simulink model "SC_FFNN_trainlm_10_10_10_10_Dec_8_M"  (R2021a)
settings: Solver=VariableStepAuto  StartTime=0.0  StopTime=35  FixedStep=0.1  MaxStep=.1  RelTol=1e-3
model workspace (MAT data in the model file):
  T = [0 0.05 0.1 0.15 0.2 0.25 0.3 0.35 0.4 0.45 0.5 0.55 ... (701 elements, 701x1)]
  U = [3.99594136536 3.99594136536 3.99594136536 3.99594136536 3.99594136536 3.99594136536 3.99594136536 3.99594136536 3.99594136536 3.99594136536 3.99594136536 3.99594136536 ... (701 elements, 701x1)]
libraries: neural x46, simulink_extras x2
(part 2 of 2)

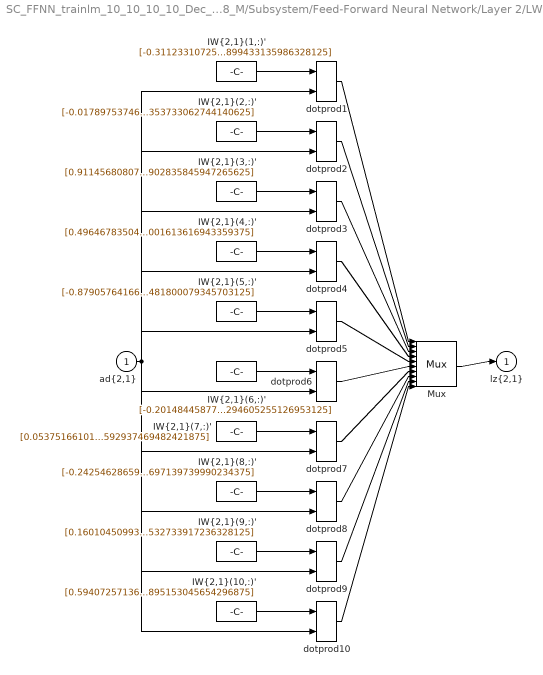
== system SC_FFNN_trainlm_10_10_10_10_Dec_8_M/Subsystem/Feed-Forward Neural Network/Layer 2/LW{2,1} ==
  "ad{2,1}" : Inport  PortDimensions=10
      mask Display: e = 0.06;c1 = [120 230 180]/255;c2 = ([120 230 180]+0)/(256+128);c3 = ([120 230 180]+128)/(256+128);patch([0 1 1 0],[0 0 1 1],c1);patch([0 1 1 1-e 1-e 0+e],[0 0 1 1-e 0+e 0+e],c2);patch([0 0 1 1-e 0+e 0+e],[0 1 1 1-e 1-e 0+e],c3);plot([0 1 1 0 0],[0 0 1 1 0]);
  "IW{2,1}(1,:)'" : Constant  Value=[-0.31123310725178632285548019353882409632205963134765625;-1.469321495607214256295947052421979606151580810546875;1.7512337188909194996000451283180154860019683837890625;-0.28837010143751540258705290398211218416690826416015625;-0.650296904248475637899673529318533837795257568359375;0.79149097122355704936325082599068991839885711669921875;-2.430225902669928217392225633375346660614013671875;-1.32538923939724639922133064828813076019287109375;-0.88929908387866252184039694839157164096832275390625;0.0617285613882530004303816895117051899433135986328125]
      mask Display: e = 0.06;c1 = [120 150 230]/255;c2 = ([120 150 230]+0)/383;c3 = ([120 150 230]+128)/383;patch([0 1 1 0],[0 0 1 1],c1);patch([0 1 1 1-e 1-e 0+e],[0 0 1 1-e 0+e 0+e],c2);patch([0 0 1 1-e 0+e 0+e],[0 1 1 1-e 1-e 0+e],c3);plot([0 1 1 0 0],[0 0 1 1 0]);disp('weights');
  "IW{2,1}(10,:)'" : Constant  Value=[0.5940725713630230497841466785757802426815032958984375;-0.2242780336341263780486343648590263910591602325439453125;1.551496659314222537062732953927479684352874755859375;-0.41231345611790548577602066870895214378833770751953125;0.20714960886964106645535821371595375239849090576171875;0.701514109569985055969709719647653400897979736328125;-0.272464453987376231669514936584164388477802276611328125;-1.03262322115372118247478283592499792575836181640625;-0.282258121891233948463906244796817190945148468017578125;0.221917317492401178213867751765064895153045654296875]
      mask Display: e = 0.06;c1 = [120 150 230]/255;c2 = ([120 150 230]+0)/383;c3 = ([120 150 230]+128)/383;patch([0 1 1 0],[0 0 1 1],c1);patch([0 1 1 1-e 1-e 0+e],[0 0 1 1-e 0+e 0+e],c2);patch([0 0 1 1-e 0+e 0+e],[0 1 1 1-e 1-e 0+e],c3);plot([0 1 1 0 0],[0 0 1 1 0]);disp('weights');
  "IW{2,1}(2,:)'" : Constant  Value=[-0.0178975374680546243932877104043654981069266796112060546875;-0.316716679552807078845688693036208860576152801513671875;0.92256475953105387954877869560732506215572357177734375;0.263275217675462636091054946518852375447750091552734375;-0.334982081241569196183860412929789163172245025634765625;0.086180170541050038490737961183185689151287078857421875;-0.2187903051905081552863663318930775858461856842041015625;1.1402682625195963428410550477565266191959381103515625;-0.69860811012117718377112396410666406154632568359375;0.3088914155141326833842185806133784353733062744140625]
      mask Display: e = 0.06;c1 = [120 150 230]/255;c2 = ([120 150 230]+0)/383;c3 = ([120 150 230]+128)/383;patch([0 1 1 0],[0 0 1 1],c1);patch([0 1 1 1-e 1-e 0+e],[0 0 1 1-e 0+e 0+e],c2);patch([0 0 1 1-e 0+e 0+e],[0 1 1 1-e 1-e 0+e],c3);plot([0 1 1 0 0],[0 0 1 1 0]);disp('weights');
  "IW{2,1}(3,:)'" : Constant  Value=[0.9114568080755713896934366857749409973621368408203125;-0.43987318638631578426867463349481113255023956298828125;-0.00022860043250971760222210737989456674768007360398769378662109375;0.2039764312835918025346160220578894950449466705322265625;1.822125124921296190905195544473826885223388671875;-0.5959660144003648962751640283386223018169403076171875;0.74163121504978324338708262075670063495635986328125;0.88662530980484632880944673161138780415058135986328125;0.384805661539336540943878617326845414936542510986328125;-0.1847616059176948599684919827268458902835845947265625]
      mask Display: e = 0.06;c1 = [120 150 230]/255;c2 = ([120 150 230]+0)/383;c3 = ([120 150 230]+128)/383;patch([0 1 1 0],[0 0 1 1],c1);patch([0 1 1 1-e 1-e 0+e],[0 0 1 1-e 0+e 0+e],c2);patch([0 0 1 1-e 0+e 0+e],[0 1 1 1-e 1-e 0+e],c3);plot([0 1 1 0 0],[0 0 1 1 0]);disp('weights');
  "IW{2,1}(4,:)'" : Constant  Value=[0.496467835040173388616580041343695484101772308349609375;0.8003342134367754656665283619076944887638092041015625;0.2715311750074949070921093152719549834728240966796875;-0.02720061211852882465667136102638323791325092315673828125;-0.127613664961616801729604731008294038474559783935546875;-0.2023171556652099967177349526537000201642513275146484375;-0.5634077333743292559375959172029979526996612548828125;-0.421629687942608855077963880830793641507625579833984375;0.1139038301844583767064023049897514283657073974609375;0.6399624455638812658975211888900958001613616943359375]
      mask Display: e = 0.06;c1 = [120 150 230]/255;c2 = ([120 150 230]+0)/383;c3 = ([120 150 230]+128)/383;patch([0 1 1 0],[0 0 1 1],c1);patch([0 1 1 1-e 1-e 0+e],[0 0 1 1-e 0+e 0+e],c2);patch([0 0 1 1-e 0+e 0+e],[0 1 1 1-e 1-e 0+e],c3);plot([0 1 1 0 0],[0 0 1 1 0]);disp('weights');
  "IW{2,1}(5,:)'" : Constant  Value=[-0.8790576416602127185484505389467813074588775634765625;-0.665663180170688040249160621897317469120025634765625;-0.46176114720288818915605588699690997600555419921875;0.396211040360616717492803218192420899868011474609375;-0.6191334656400917513252579738036729395389556884765625;-0.0359558779362874059160049000638537108898162841796875;0.64875253337767002648206471349112689495086669921875;0.1887125013286616859176092475536279380321502685546875;0.39189862660321583831546377041377127170562744140625;0.436717886411767342025314064812846481800079345703125]
      mask Display: e = 0.06;c1 = [120 150 230]/255;c2 = ([120 150 230]+0)/383;c3 = ([120 150 230]+128)/383;patch([0 1 1 0],[0 0 1 1],c1);patch([0 1 1 1-e 1-e 0+e],[0 0 1 1-e 0+e 0+e],c2);patch([0 0 1 1-e 0+e 0+e],[0 1 1 1-e 1-e 0+e],c3);plot([0 1 1 0 0],[0 0 1 1 0]);disp('weights');
  "IW{2,1}(6,:)'" : Constant  Value=[-0.2014844587728485958422197654726915061473846435546875;-0.7875673101426723388129857994499616324901580810546875;-0.1543287699823843173163595565711148083209991455078125;0.3330558268051737602633011192665435373783111572265625;-0.2621669078722101975387204220169223845005035400390625;-0.7587767734056753976545905970851890742778778076171875;0.9653267994439005406093201600015163421630859375;-0.9549748145195364745774213588447310030460357666015625;0.3997756998565831221270627793273888528347015380859375;0.93729866046218734965123076108284294605255126953125]
      mask Display: e = 0.06;c1 = [120 150 230]/255;c2 = ([120 150 230]+0)/383;c3 = ([120 150 230]+128)/383;patch([0 1 1 0],[0 0 1 1],c1);patch([0 1 1 1-e 1-e 0+e],[0 0 1 1-e 0+e 0+e],c2);patch([0 0 1 1-e 0+e 0+e],[0 1 1 1-e 1-e 0+e],c3);plot([0 1 1 0 0],[0 0 1 1 0]);disp('weights');
  "IW{2,1}(7,:)'" : Constant  Value=[0.05375166101659178963245722115971148014068603515625;-0.869132604652068874173664880800060927867889404296875;0.0957418024296894376590216779732145369052886962890625;-0.643735091199324482857946350122801959514617919921875;-0.4580628093162031344576234914711676537990570068359375;0.17901496939011796172280810424126684665679931640625;-0.509974934208484054209975511184893548488616943359375;-1.52191856716526974224734658491797745227813720703125;-0.02185677440340805244289867914631031453609466552734375;0.0626678131313489483744660901720635592937469482421875]
      mask Display: e = 0.06;c1 = [120 150 230]/255;c2 = ([120 150 230]+0)/383;c3 = ([120 150 230]+128)/383;patch([0 1 1 0],[0 0 1 1],c1);patch([0 1 1 1-e 1-e 0+e],[0 0 1 1-e 0+e 0+e],c2);patch([0 0 1 1-e 0+e 0+e],[0 1 1 1-e 1-e 0+e],c3);plot([0 1 1 0 0],[0 0 1 1 0]);disp('weights');
  "IW{2,1}(8,:)'" : Constant  Value=[-0.2425462865928274813764886630451655946671962738037109375;-0.60067130915694288972872527665458619594573974609375;1.0197024905286109497382085464778356254100799560546875;-0.60109024079500006365606168401427567005157470703125;1.095065618142897267972557528992183506488800048828125;-0.79903802226295683741597031257697381079196929931640625;-0.4110697480527376601600053618312813341617584228515625;-0.81563251092069199987832917031482793390750885009765625;-0.91728451490253515299144737582537345588207244873046875;-0.349708636358879942918065353296697139739990234375]
      mask Display: e = 0.06;c1 = [120 150 230]/255;c2 = ([120 150 230]+0)/383;c3 = ([120 150 230]+128)/383;patch([0 1 1 0],[0 0 1 1],c1);patch([0 1 1 1-e 1-e 0+e],[0 0 1 1-e 0+e 0+e],c2);patch([0 0 1 1-e 0+e 0+e],[0 1 1 1-e 1-e 0+e],c3);plot([0 1 1 0 0],[0 0 1 1 0]);disp('weights');
  "IW{2,1}(9,:)'" : Constant  Value=[0.1601045099351747491578379367638262920081615447998046875;-0.0206247239679522298416713965707458555698394775390625;-0.3703365745029938427279603274655528366565704345703125;0.8496229838840345660599950861069373786449432373046875;-0.726008181683521769400613266043365001678466796875;-0.34248857917064590150602043649996630847454071044921875;0.1681386665569040150813862055656500160694122314453125;-0.632527844483548040699361081351526081562042236328125;-0.862387801763897510198830786976031959056854248046875;-0.7887415933419561486772408898104913532733917236328125]
      mask Display: e = 0.06;c1 = [120 150 230]/255;c2 = ([120 150 230]+0)/383;c3 = ([120 150 230]+128)/383;patch([0 1 1 0],[0 0 1 1],c1);patch([0 1 1 1-e 1-e 0+e],[0 0 1 1-e 0+e 0+e],c2);patch([0 0 1 1-e 0+e 0+e],[0 1 1 1-e 1-e 0+e],c3);plot([0 1 1 0 0],[0 0 1 1 0]);disp('weights');
  Mux : Mux  Inputs=10
      mask Display: e = 0.06;c1 = [120 150 230]/255;c2 = ([120 150 230]+0)/383;c3 = ([120 150 230]+128)/383;patch([0 1 1 0],[0 0 1 1],c1);patch([0 1 1 1-e 1-e 0+e],[0 0 1 1-e 0+e 0+e],c2);patch([0 0 1 1-e 0+e 0+e],[0 1 1 1-e 1-e 0+e],c3);plot([0 1 1 0 0],[0 0 1 1 0]);disp('Mux');
  dotprod{1..10} (10 alike) : neural/Weight Functions/dotprod
  "lz{2,1}" : Outport
      mask Display: e = 0.06;c1 = [120 230 180]/255;c2 = ([120 230 180]+0)/(256+128);c3 = ([120 230 180]+128)/(256+128);patch([0 1 1 0],[0 0 1 1],c1);patch([0 1 1 1-e 1-e 0+e],[0 0 1 1-e 0+e 0+e],c2);patch([0 0 1 1-e 0+e 0+e],[0 1 1 1-e 1-e 0+e],c3);plot([0 1 1 0 0],[0 0 1 1 0]);
  wires:
  "IW{2,1}(1,:)'"/1 -> dotprod1/1
  "ad{2,1}"/1 -> dotprod1/2, dotprod2/2, dotprod3/2, dotprod4/2, dotprod5/2, dotprod6/2, dotprod7/2, dotprod8/2, dotprod9/2, dotprod10/2
  dotprod1/1 -> Mux/1
  "IW{2,1}(2,:)'"/1 -> dotprod2/1
  dotprod2/1 -> Mux/2
  "IW{2,1}(3,:)'"/1 -> dotprod3/1
  dotprod3/1 -> Mux/3
  "IW{2,1}(4,:)'"/1 -> dotprod4/1
  dotprod4/1 -> Mux/4
  "IW{2,1}(5,:)'"/1 -> dotprod5/1
  dotprod5/1 -> Mux/5
  "IW{2,1}(6,:)'"/1 -> dotprod6/1
  dotprod6/1 -> Mux/6
  "IW{2,1}(7,:)'"/1 -> dotprod7/1
  dotprod7/1 -> Mux/7
  "IW{2,1}(8,:)'"/1 -> dotprod8/1
  dotprod8/1 -> Mux/8
  "IW{2,1}(9,:)'"/1 -> dotprod9/1
  dotprod9/1 -> Mux/9
  "IW{2,1}(10,:)'"/1 -> dotprod10/1
  dotprod10/1 -> Mux/10
  Mux/1 -> "lz{2,1}"/1

== system SC_FFNN_trainlm_10_10_10_10_Dec_8_M/Subsystem/Feed-Forward Neural Network/Layer 3/Delays 1 ==
  "p{3}" : Inport  PortDimensions=10
      mask Display: e = 0.06;c1 = [120 230 180]/255;c2 = ([120 230 180]+0)/(256+128);c3 = ([120 230 180]+128)/(256+128);patch([0 1 1 0],[0 0 1 1],c1);patch([0 1 1 1-e 1-e 0+e],[0 0 1 1-e 0+e 0+e],c2);patch([0 0 1 1-e 0+e 0+e],[0 1 1 1-e 1-e 0+e],c3);plot([0 1 1 0 0],[0 0 1 1 0]);
  mux : Mux  Inputs=1
      mask Display: e = 0.06;c1 = [120 150 230]/255;c2 = ([120 150 230]+0)/383;c3 = ([120 150 230]+128)/383;patch([0 1 1 0],[0 0 1 1],c1);patch([0 1 1 1-e 1-e 0+e],[0 0 1 1-e 0+e 0+e],c2);patch([0 0 1 1-e 0+e 0+e],[0 1 1 1-e 1-e 0+e],c3);plot([0 1 1 0 0],[0 0 1 1 0]);disp('Mux')
  "pd{3,2}" : Outport
      mask Display: e = 0.06;c1 = [120 230 180]/255;c2 = ([120 230 180]+0)/(256+128);c3 = ([120 230 180]+128)/(256+128);patch([0 1 1 0],[0 0 1 1],c1);patch([0 1 1 1-e 1-e 0+e],[0 0 1 1-e 0+e 0+e],c2);patch([0 0 1 1-e 0+e 0+e],[0 1 1 1-e 1-e 0+e],c3);plot([0 1 1 0 0],[0 0 1 1 0]);
  wires:
  "p{3}"/1 -> mux/1
  mux/1 -> "pd{3,2}"/1

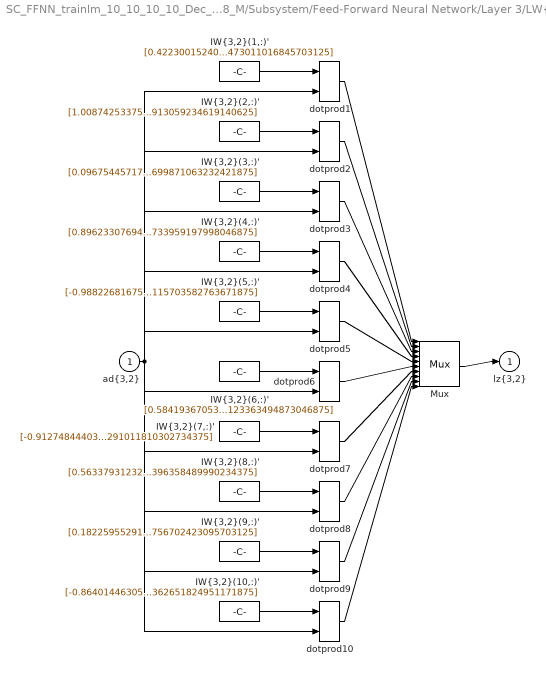
== system SC_FFNN_trainlm_10_10_10_10_Dec_8_M/Subsystem/Feed-Forward Neural Network/Layer 3/LW{3,2} ==
  "ad{3,2}" : Inport  PortDimensions=10
      mask Display: e = 0.06;c1 = [120 230 180]/255;c2 = ([120 230 180]+0)/(256+128);c3 = ([120 230 180]+128)/(256+128);patch([0 1 1 0],[0 0 1 1],c1);patch([0 1 1 1-e 1-e 0+e],[0 0 1 1-e 0+e 0+e],c2);patch([0 0 1 1-e 0+e 0+e],[0 1 1 1-e 1-e 0+e],c3);plot([0 1 1 0 0],[0 0 1 1 0]);
  "IW{3,2}(1,:)'" : Constant  Value=[0.42230015240333396153715739274048246443271636962890625;-0.464755181849058229825999433160177432000637054443359375;1.9453528874502861167883338566753081977367401123046875;-0.32490527135295133032144576645805500447750091552734375;-0.4618768266279633660786885229754261672496795654296875;0.295235260345368732970428027329035103321075439453125;0.00822064630778608640415683339597308076918125152587890625;1.236309731525776722804721430293284356594085693359375;0.089432221053525662313177235773764550685882568359375;-0.39772990518832440631769031824660487473011016845703125]
      mask Display: e = 0.06;c1 = [120 150 230]/255;c2 = ([120 150 230]+0)/383;c3 = ([120 150 230]+128)/383;patch([0 1 1 0],[0 0 1 1],c1);patch([0 1 1 1-e 1-e 0+e],[0 0 1 1-e 0+e 0+e],c2);patch([0 0 1 1-e 0+e 0+e],[0 1 1 1-e 1-e 0+e],c3);plot([0 1 1 0 0],[0 0 1 1 0]);disp('weights');
  "IW{3,2}(10,:)'" : Constant  Value=[-0.8640144630599788655445081531070172786712646484375;-0.2264576109580307416990763158537447452545166015625;-0.92847453346176411770329650607891380786895751953125;0.834848684098764781680301894084550440311431884765625;0.288885562862672973238886697799898684024810791015625;-0.0997246060682079882298012307728640735149383544921875;0.226921473625750547142843061010353267192840576171875;0.27863392208021675600093658431433141231536865234375;-0.872817258049788602392027314635924994945526123046875;-0.7222515943416893957618185595492832362651824951171875]
      mask Display: e = 0.06;c1 = [120 150 230]/255;c2 = ([120 150 230]+0)/383;c3 = ([120 150 230]+128)/383;patch([0 1 1 0],[0 0 1 1],c1);patch([0 1 1 1-e 1-e 0+e],[0 0 1 1-e 0+e 0+e],c2);patch([0 0 1 1-e 0+e 0+e],[0 1 1 1-e 1-e 0+e],c3);plot([0 1 1 0 0],[0 0 1 1 0]);disp('weights');
  "IW{3,2}(2,:)'" : Constant  Value=[1.0087425337536386482639727546484209597110748291015625;-0.620528400869083451851793142850510776042938232421875;-0.63207781154537900913936709912377409636974334716796875;0.443516066782204898544250681879930198192596435546875;0.5310000332428768121673101632040925323963165283203125;0.3580335081864038926369175896979868412017822265625;0.3238895038113038804539201009902171790599822998046875;0.195282319319245944999607900172122754156589508056640625;0.29462296058625536687713974970392882823944091796875;0.40906652213958738517618485275306738913059234619140625]
      mask Display: e = 0.06;c1 = [120 150 230]/255;c2 = ([120 150 230]+0)/383;c3 = ([120 150 230]+128)/383;patch([0 1 1 0],[0 0 1 1],c1);patch([0 1 1 1-e 1-e 0+e],[0 0 1 1-e 0+e 0+e],c2);patch([0 0 1 1-e 0+e 0+e],[0 1 1 1-e 1-e 0+e],c3);plot([0 1 1 0 0],[0 0 1 1 0]);disp('weights');
  "IW{3,2}(3,:)'" : Constant  Value=[0.09675445717161339220790949866568553261458873748779296875;0.1346160128529440280775730798268341459333896636962890625;-0.08934636093222021735460458558009122498333454132080078125;0.1238463946215047906118655873797251842916011810302734375;-0.6226760464170180142673416412435472011566162109375;0.2715734210281672833531274591223336756229400634765625;0.51223817361442025575257730451994575560092926025390625;0.224710267556270049116307063741260208189487457275390625;0.1367654806136633371949073989526368677616119384765625;-0.82036806334343104207817987116868607699871063232421875]
      mask Display: e = 0.06;c1 = [120 150 230]/255;c2 = ([120 150 230]+0)/383;c3 = ([120 150 230]+128)/383;patch([0 1 1 0],[0 0 1 1],c1);patch([0 1 1 1-e 1-e 0+e],[0 0 1 1-e 0+e 0+e],c2);patch([0 0 1 1-e 0+e 0+e],[0 1 1 1-e 1-e 0+e],c3);plot([0 1 1 0 0],[0 0 1 1 0]);disp('weights');
  "IW{3,2}(4,:)'" : Constant  Value=[0.8962330769412141240337632552837021648883819580078125;0.206166966535160367524071034495136700570583343505859375;0.06339036844936292436347713419309002347290515899658203125;-0.298873791997468496450807151632034219801425933837890625;-0.425003653867737529736814394709654152393341064453125;0.890348226218802718534561790875159204006195068359375;-0.4335997277560432738852114198380149900913238525390625;-0.06458350428076327365278785919144866056740283966064453125;0.55489992620035233361619475545012392103672027587890625;0.93451149416491741117596347976359538733959197998046875]
      mask Display: e = 0.06;c1 = [120 150 230]/255;c2 = ([120 150 230]+0)/383;c3 = ([120 150 230]+128)/383;patch([0 1 1 0],[0 0 1 1],c1);patch([0 1 1 1-e 1-e 0+e],[0 0 1 1-e 0+e 0+e],c2);patch([0 0 1 1-e 0+e 0+e],[0 1 1 1-e 1-e 0+e],c3);plot([0 1 1 0 0],[0 0 1 1 0]);disp('weights');
  "IW{3,2}(5,:)'" : Constant  Value=[-0.9882268167530396940634318525553680956363677978515625;-0.8243020120842292630669589925673790276050567626953125;-0.474056250874433426911735978137585334479808807373046875;-0.3177507859017814073609997649327851831912994384765625;-0.81777307262693010869725185330025851726531982421875;-0.582130155147954297945034340955317020416259765625;0.273352384266664583112316222468507476150989532470703125;-0.421602895088965812231407426224905066192150115966796875;0.0449906115542042517319032413070090115070343017578125;0.137525390869700003815268019025097601115703582763671875]
      mask Display: e = 0.06;c1 = [120 150 230]/255;c2 = ([120 150 230]+0)/383;c3 = ([120 150 230]+128)/383;patch([0 1 1 0],[0 0 1 1],c1);patch([0 1 1 1-e 1-e 0+e],[0 0 1 1-e 0+e 0+e],c2);patch([0 0 1 1-e 0+e 0+e],[0 1 1 1-e 1-e 0+e],c3);plot([0 1 1 0 0],[0 0 1 1 0]);disp('weights');
  "IW{3,2}(6,:)'" : Constant  Value=[0.58419367053035198278365669466438703238964080810546875;0.90251141886128272151523788124904967844486236572265625;0.62012722071280867996989627499715425074100494384765625;0.2184737737019071257549285292043350636959075927734375;0.1524187613260139517734614855726249516010284423828125;0.4185634054210896071168690468766726553440093994140625;-0.1364832995021457995310498745311633683741092681884765625;-0.9555699724308206466361070852144621312618255615234375;0.96741393758073634945304775101249106228351593017578125;0.162645047395365505149555929165217094123363494873046875]
      mask Display: e = 0.06;c1 = [120 150 230]/255;c2 = ([120 150 230]+0)/383;c3 = ([120 150 230]+128)/383;patch([0 1 1 0],[0 0 1 1],c1);patch([0 1 1 1-e 1-e 0+e],[0 0 1 1-e 0+e 0+e],c2);patch([0 0 1 1-e 0+e 0+e],[0 1 1 1-e 1-e 0+e],c3);plot([0 1 1 0 0],[0 0 1 1 0]);disp('weights');
  "IW{3,2}(7,:)'" : Constant  Value=[-0.912748444038607775752325323992408812046051025390625;-0.0834190636841314614446929454061319120228290557861328125;-0.31333242893386803462618672710959799587726593017578125;-0.380566736422279283669212190943653695285320281982421875;0.366726486589306066576909870491363108158111572265625;-0.5275388460124068590317847338155843317508697509765625;0.6838583053826179369849569411599077284336090087890625;0.8736203018612906934237116729491390287876129150390625;-0.507482918142163175190262336400337517261505126953125;0.78501189835875118117058946154429577291011810302734375]
      mask Display: e = 0.06;c1 = [120 150 230]/255;c2 = ([120 150 230]+0)/383;c3 = ([120 150 230]+128)/383;patch([0 1 1 0],[0 0 1 1],c1);patch([0 1 1 1-e 1-e 0+e],[0 0 1 1-e 0+e 0+e],c2);patch([0 0 1 1-e 0+e 0+e],[0 1 1 1-e 1-e 0+e],c3);plot([0 1 1 0 0],[0 0 1 1 0]);disp('weights');
  "IW{3,2}(8,:)'" : Constant  Value=[0.563379312328809334076140657998621463775634765625;-1.418848345873518379534061750746332108974456787109375;-0.063815894302275300020710346871055662631988525390625;1.146209905486756497339229099452495574951171875;0.0931862291806455633746963940211571753025054931640625;-0.7612075044053889794071210417314432561397552490234375;0.521565268594802677881716590491123497486114501953125;0.0301695998231464035388427191719529218971729278564453125;-0.61431491299480345258388069851207546889781951904296875;1.5400529863936875951679894569679163396358489990234375]
      mask Display: e = 0.06;c1 = [120 150 230]/255;c2 = ([120 150 230]+0)/383;c3 = ([120 150 230]+128)/383;patch([0 1 1 0],[0 0 1 1],c1);patch([0 1 1 1-e 1-e 0+e],[0 0 1 1-e 0+e 0+e],c2);patch([0 0 1 1-e 0+e 0+e],[0 1 1 1-e 1-e 0+e],c3);plot([0 1 1 0 0],[0 0 1 1 0]);disp('weights');
  "IW{3,2}(9,:)'" : Constant  Value=[0.1822595529134967140549861142062582075595855712890625;-0.3018214640064897924531805983860976994037628173828125;-0.496998609737553553866717948039877228438854217529296875;-0.52541831536877270369956249851384200155735015869140625;-0.1485423162576242628318823335575871169567108154296875;0.21460788137126929342457515303976833820343017578125;-0.53612257790433714976785495309741236269474029541015625;-0.080908169545872710148870510238339193165302276611328125;-0.7806050709536116460895982527290470898151397705078125;-0.437291746960222493800785059647751040756702423095703125]
      mask Display: e = 0.06;c1 = [120 150 230]/255;c2 = ([120 150 230]+0)/383;c3 = ([120 150 230]+128)/383;patch([0 1 1 0],[0 0 1 1],c1);patch([0 1 1 1-e 1-e 0+e],[0 0 1 1-e 0+e 0+e],c2);patch([0 0 1 1-e 0+e 0+e],[0 1 1 1-e 1-e 0+e],c3);plot([0 1 1 0 0],[0 0 1 1 0]);disp('weights');
  Mux : Mux  Inputs=10
      mask Display: e = 0.06;c1 = [120 150 230]/255;c2 = ([120 150 230]+0)/383;c3 = ([120 150 230]+128)/383;patch([0 1 1 0],[0 0 1 1],c1);patch([0 1 1 1-e 1-e 0+e],[0 0 1 1-e 0+e 0+e],c2);patch([0 0 1 1-e 0+e 0+e],[0 1 1 1-e 1-e 0+e],c3);plot([0 1 1 0 0],[0 0 1 1 0]);disp('Mux');
  dotprod{1..10} (10 alike) : neural/Weight Functions/dotprod
  "lz{3,2}" : Outport
      mask Display: e = 0.06;c1 = [120 230 180]/255;c2 = ([120 230 180]+0)/(256+128);c3 = ([120 230 180]+128)/(256+128);patch([0 1 1 0],[0 0 1 1],c1);patch([0 1 1 1-e 1-e 0+e],[0 0 1 1-e 0+e 0+e],c2);patch([0 0 1 1-e 0+e 0+e],[0 1 1 1-e 1-e 0+e],c3);plot([0 1 1 0 0],[0 0 1 1 0]);
  wires:
  "IW{3,2}(1,:)'"/1 -> dotprod1/1
  "ad{3,2}"/1 -> dotprod1/2, dotprod2/2, dotprod3/2, dotprod4/2, dotprod5/2, dotprod6/2, dotprod7/2, dotprod8/2, dotprod9/2, dotprod10/2
  dotprod1/1 -> Mux/1
  "IW{3,2}(2,:)'"/1 -> dotprod2/1
  dotprod2/1 -> Mux/2
  "IW{3,2}(3,:)'"/1 -> dotprod3/1
  dotprod3/1 -> Mux/3
  "IW{3,2}(4,:)'"/1 -> dotprod4/1
  dotprod4/1 -> Mux/4
  "IW{3,2}(5,:)'"/1 -> dotprod5/1
  dotprod5/1 -> Mux/5
  "IW{3,2}(6,:)'"/1 -> dotprod6/1
  dotprod6/1 -> Mux/6
  "IW{3,2}(7,:)'"/1 -> dotprod7/1
  dotprod7/1 -> Mux/7
  "IW{3,2}(8,:)'"/1 -> dotprod8/1
  dotprod8/1 -> Mux/8
  "IW{3,2}(9,:)'"/1 -> dotprod9/1
  dotprod9/1 -> Mux/9
  "IW{3,2}(10,:)'"/1 -> dotprod10/1
  dotprod10/1 -> Mux/10
  Mux/1 -> "lz{3,2}"/1

== system SC_FFNN_trainlm_10_10_10_10_Dec_8_M/Subsystem/Feed-Forward Neural Network/Layer 4/Delays 1 ==
  "p{4}" : Inport  PortDimensions=10
      mask Display: e = 0.06;c1 = [120 230 180]/255;c2 = ([120 230 180]+0)/(256+128);c3 = ([120 230 180]+128)/(256+128);patch([0 1 1 0],[0 0 1 1],c1);patch([0 1 1 1-e 1-e 0+e],[0 0 1 1-e 0+e 0+e],c2);patch([0 0 1 1-e 0+e 0+e],[0 1 1 1-e 1-e 0+e],c3);plot([0 1 1 0 0],[0 0 1 1 0]);
  mux : Mux  Inputs=1
      mask Display: e = 0.06;c1 = [120 150 230]/255;c2 = ([120 150 230]+0)/383;c3 = ([120 150 230]+128)/383;patch([0 1 1 0],[0 0 1 1],c1);patch([0 1 1 1-e 1-e 0+e],[0 0 1 1-e 0+e 0+e],c2);patch([0 0 1 1-e 0+e 0+e],[0 1 1 1-e 1-e 0+e],c3);plot([0 1 1 0 0],[0 0 1 1 0]);disp('Mux')
  "pd{4,3}" : Outport
      mask Display: e = 0.06;c1 = [120 230 180]/255;c2 = ([120 230 180]+0)/(256+128);c3 = ([120 230 180]+128)/(256+128);patch([0 1 1 0],[0 0 1 1],c1);patch([0 1 1 1-e 1-e 0+e],[0 0 1 1-e 0+e 0+e],c2);patch([0 0 1 1-e 0+e 0+e],[0 1 1 1-e 1-e 0+e],c3);plot([0 1 1 0 0],[0 0 1 1 0]);
  wires:
  "p{4}"/1 -> mux/1
  mux/1 -> "pd{4,3}"/1

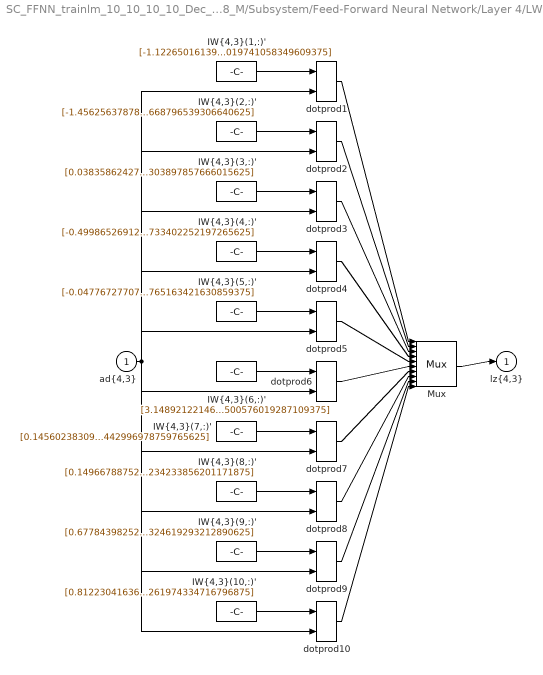
== system SC_FFNN_trainlm_10_10_10_10_Dec_8_M/Subsystem/Feed-Forward Neural Network/Layer 4/LW{4,3} ==
  "ad{4,3}" : Inport  PortDimensions=10
      mask Display: e = 0.06;c1 = [120 230 180]/255;c2 = ([120 230 180]+0)/(256+128);c3 = ([120 230 180]+128)/(256+128);patch([0 1 1 0],[0 0 1 1],c1);patch([0 1 1 1-e 1-e 0+e],[0 0 1 1-e 0+e 0+e],c2);patch([0 0 1 1-e 0+e 0+e],[0 1 1 1-e 1-e 0+e],c3);plot([0 1 1 0 0],[0 0 1 1 0]);
  "IW{4,3}(1,:)'" : Constant  Value=[-1.12265016139534079542272593243978917598724365234375;0.4726801486024034826272099962807260453701019287109375;0.36268289823253230252930734422989189624786376953125;0.10701181538384048341772114554260042496025562286376953125;-0.1757047340874803020849270751568838022649288177490234375;-0.410743175435414276108758713235147297382354736328125;0.7619926248164741178214853789540939033031463623046875;-0.0160515639463252000884718739825984812341630458831787109375;0.108546340217925696425282922064070589840412139892578125;0.5380581706717924017624454791075550019741058349609375]
      mask Display: e = 0.06;c1 = [120 150 230]/255;c2 = ([120 150 230]+0)/383;c3 = ([120 150 230]+128)/383;patch([0 1 1 0],[0 0 1 1],c1);patch([0 1 1 1-e 1-e 0+e],[0 0 1 1-e 0+e 0+e],c2);patch([0 0 1 1-e 0+e 0+e],[0 1 1 1-e 1-e 0+e],c3);plot([0 1 1 0 0],[0 0 1 1 0]);disp('weights');
  "IW{4,3}(10,:)'" : Constant  Value=[0.81223041636448922719893062094342894852161407470703125;-0.6299144486870582593240897040232084691524505615234375;-0.47363046330215030632615480499225668609142303466796875;1.27974104111037689790464355610311031341552734375;-0.3162884489577117985703580416156910359859466552734375;-0.26994773324075749254546963129541836678981781005859375;0.37255391979251373246739831301965750753879547119140625;1.2058349720824121931173067423515021800994873046875;1.1774657306357223518489263369701802730560302734375;-0.581189831958130564970588238793425261974334716796875]
      mask Display: e = 0.06;c1 = [120 150 230]/255;c2 = ([120 150 230]+0)/383;c3 = ([120 150 230]+128)/383;patch([0 1 1 0],[0 0 1 1],c1);patch([0 1 1 1-e 1-e 0+e],[0 0 1 1-e 0+e 0+e],c2);patch([0 0 1 1-e 0+e 0+e],[0 1 1 1-e 1-e 0+e],c3);plot([0 1 1 0 0],[0 0 1 1 0]);disp('weights');
  "IW{4,3}(2,:)'" : Constant  Value=[-1.456256378784395177916621832991950213909149169921875;-0.1386526565771135366400557131782989017665386199951171875;-0.39803847560947247519180791641701944172382354736328125;0.376741990868013854054652256309054791927337646484375;0.5886370628508659219590981592773459851741790771484375;-1.3007377607374117634009280664031393826007843017578125;0.044241393079879183514169227464662981219589710235595703125;0.89068970193047025674104588688351213932037353515625;-0.15236701106996985988217829799395985901355743408203125;0.162892975750795532263737186440266668796539306640625]
      mask Display: e = 0.06;c1 = [120 150 230]/255;c2 = ([120 150 230]+0)/383;c3 = ([120 150 230]+128)/383;patch([0 1 1 0],[0 0 1 1],c1);patch([0 1 1 1-e 1-e 0+e],[0 0 1 1-e 0+e 0+e],c2);patch([0 0 1 1-e 0+e 0+e],[0 1 1 1-e 1-e 0+e],c3);plot([0 1 1 0 0],[0 0 1 1 0]);disp('weights');
  "IW{4,3}(3,:)'" : Constant  Value=[0.0383586242768238216971354859197163023054599761962890625;0.366831733935956805225941934622824192047119140625;0.6813027073797972565927238974836654961109161376953125;-0.49480183953733070101321800393634475767612457275390625;0.1760521106169949945297048543579876422882080078125;-0.66191523986713407534665520870476029813289642333984375;0.77325633438717866763312258626683615148067474365234375;-0.60278208424459089886937590563320554792881011962890625;-0.5065309480280502096860573146841488778591156005859375;0.856626124628375951175485170097090303897857666015625]
      mask Display: e = 0.06;c1 = [120 150 230]/255;c2 = ([120 150 230]+0)/383;c3 = ([120 150 230]+128)/383;patch([0 1 1 0],[0 0 1 1],c1);patch([0 1 1 1-e 1-e 0+e],[0 0 1 1-e 0+e 0+e],c2);patch([0 0 1 1-e 0+e 0+e],[0 1 1 1-e 1-e 0+e],c3);plot([0 1 1 0 0],[0 0 1 1 0]);disp('weights');
  "IW{4,3}(4,:)'" : Constant  Value=[-0.499865269128736688930558784704771824181079864501953125;0.42112596405173430280655111346277408301830291748046875;-0.1813874941957727970898162084267823956906795501708984375;0.451995454503296312243065813163411803543567657470703125;-0.6655677214106654471237334291799925267696380615234375;-0.415036093549412565817391396194580011069774627685546875;0.59214694555344415949349468064610846340656280517578125;-0.0368443626356440845359685454241116531193256378173828125;0.380526402522060547273241581933689303696155548095703125;0.1601807315168832790419628508971072733402252197265625]
      mask Display: e = 0.06;c1 = [120 150 230]/255;c2 = ([120 150 230]+0)/383;c3 = ([120 150 230]+128)/383;patch([0 1 1 0],[0 0 1 1],c1);patch([0 1 1 1-e 1-e 0+e],[0 0 1 1-e 0+e 0+e],c2);patch([0 0 1 1-e 0+e 0+e],[0 1 1 1-e 1-e 0+e],c3);plot([0 1 1 0 0],[0 0 1 1 0]);disp('weights');
  "IW{4,3}(5,:)'" : Constant  Value=[-0.04776727707786297683067999741979292593896389007568359375;0.0106023646572297840229293086622419650666415691375732421875;0.497730739226063756408535709852003492414951324462890625;0.72241584896026811435376657755114138126373291015625;-0.6002743542850959013179590328945778310298919677734375;1.2088103282487951961599037531414069235324859619140625;-0.02485874553842122580693541067375917918980121612548828125;1.5011062275827795620131155374110676348209381103515625;-0.5390709148934271777164894956513307988643646240234375;-0.96603412332547744512112330994568765163421630859375]
      mask Display: e = 0.06;c1 = [120 150 230]/255;c2 = ([120 150 230]+0)/383;c3 = ([120 150 230]+128)/383;patch([0 1 1 0],[0 0 1 1],c1);patch([0 1 1 1-e 1-e 0+e],[0 0 1 1-e 0+e 0+e],c2);patch([0 0 1 1-e 0+e 0+e],[0 1 1 1-e 1-e 0+e],c3);plot([0 1 1 0 0],[0 0 1 1 0]);disp('weights');
  "IW{4,3}(6,:)'" : Constant  Value=[3.14892122146403607985121197998523712158203125;-0.9781958684821179250690192930051125586032867431640625;-0.1161308596180801455677311651015770621597766876220703125;0.1233693019945746593979407634833478368818759918212890625;-0.1663410627215382853183456290935282595455646514892578125;0.79995812152368783731759549482376314699649810791015625;0.93639556448059835247477167285978794097900390625;1.1269111904835689141890497921849600970745086669921875;0.33816517950124824753999064341769553720951080322265625;-0.7582808578028836787865429869270883500576019287109375]
      mask Display: e = 0.06;c1 = [120 150 230]/255;c2 = ([120 150 230]+0)/383;c3 = ([120 150 230]+128)/383;patch([0 1 1 0],[0 0 1 1],c1);patch([0 1 1 1-e 1-e 0+e],[0 0 1 1-e 0+e 0+e],c2);patch([0 0 1 1-e 0+e 0+e],[0 1 1 1-e 1-e 0+e],c3);plot([0 1 1 0 0],[0 0 1 1 0]);disp('weights');
  "IW{4,3}(7,:)'" : Constant  Value=[0.145602383097704624059787192891235463321208953857421875;-0.364405337822077346476845605138805694878101348876953125;0.82318577205773824090329071623273193836212158203125;0.52140036778095322222981167215039022266864776611328125;0.6103466701085229484391447840607725083827972412109375;-0.392161108531997371073885005898773670196533203125;0.717693122595087107384870250825770199298858642578125;0.2496333928149794545436890302880783565342426300048828125;0.531203091863486687174145117751322686672210693359375;0.725421437399339286145050209597684442996978759765625]
      mask Display: e = 0.06;c1 = [120 150 230]/255;c2 = ([120 150 230]+0)/383;c3 = ([120 150 230]+128)/383;patch([0 1 1 0],[0 0 1 1],c1);patch([0 1 1 1-e 1-e 0+e],[0 0 1 1-e 0+e 0+e],c2);patch([0 0 1 1-e 0+e 0+e],[0 1 1 1-e 1-e 0+e],c3);plot([0 1 1 0 0],[0 0 1 1 0]);disp('weights');
  "IW{4,3}(8,:)'" : Constant  Value=[0.1496678875255581520065106815309263765811920166015625;-0.2131730131059011157379501355535467155277729034423828125;0.427568728602545300443438236470683477818965911865234375;-0.39622974342622330201635350022115744650363922119140625;0.6511676315723111674316214703139849007129669189453125;0.2207861180709015658241156643271096982061862945556640625;1.2010481055241661874077863103593699634075164794921875;0.96409085727123267073324086595675908029079437255859375;0.426418643526723595282845735709997825324535369873046875;-0.031406977575795025359184364788234233856201171875]
      mask Display: e = 0.06;c1 = [120 150 230]/255;c2 = ([120 150 230]+0)/383;c3 = ([120 150 230]+128)/383;patch([0 1 1 0],[0 0 1 1],c1);patch([0 1 1 1-e 1-e 0+e],[0 0 1 1-e 0+e 0+e],c2);patch([0 0 1 1-e 0+e 0+e],[0 1 1 1-e 1-e 0+e],c3);plot([0 1 1 0 0],[0 0 1 1 0]);disp('weights');
  "IW{4,3}(9,:)'" : Constant  Value=[0.67784398252901578718621067309868521988391876220703125;-0.5552409488232845635735657197074033319950103759765625;-0.198957701411829945836728938957094214856624603271484375;0.70026315407700312487548899298417381942272186279296875;0.6024883798819538061053435740177519619464874267578125;-1.039184519328525624359826906584203243255615234375;-1.0389325176084234225726277145440690219402313232421875;0.65128119690307784139804425649344921112060546875;0.8735504237166347163423552046879194676876068115234375;0.6897113491525264095116654061712324619293212890625]
      mask Display: e = 0.06;c1 = [120 150 230]/255;c2 = ([120 150 230]+0)/383;c3 = ([120 150 230]+128)/383;patch([0 1 1 0],[0 0 1 1],c1);patch([0 1 1 1-e 1-e 0+e],[0 0 1 1-e 0+e 0+e],c2);patch([0 0 1 1-e 0+e 0+e],[0 1 1 1-e 1-e 0+e],c3);plot([0 1 1 0 0],[0 0 1 1 0]);disp('weights');
  Mux : Mux  Inputs=10
      mask Display: e = 0.06;c1 = [120 150 230]/255;c2 = ([120 150 230]+0)/383;c3 = ([120 150 230]+128)/383;patch([0 1 1 0],[0 0 1 1],c1);patch([0 1 1 1-e 1-e 0+e],[0 0 1 1-e 0+e 0+e],c2);patch([0 0 1 1-e 0+e 0+e],[0 1 1 1-e 1-e 0+e],c3);plot([0 1 1 0 0],[0 0 1 1 0]);disp('Mux');
  dotprod{1..10} (10 alike) : neural/Weight Functions/dotprod
  "lz{4,3}" : Outport
      mask Display: e = 0.06;c1 = [120 230 180]/255;c2 = ([120 230 180]+0)/(256+128);c3 = ([120 230 180]+128)/(256+128);patch([0 1 1 0],[0 0 1 1],c1);patch([0 1 1 1-e 1-e 0+e],[0 0 1 1-e 0+e 0+e],c2);patch([0 0 1 1-e 0+e 0+e],[0 1 1 1-e 1-e 0+e],c3);plot([0 1 1 0 0],[0 0 1 1 0]);
  wires:
  "IW{4,3}(1,:)'"/1 -> dotprod1/1
  "ad{4,3}"/1 -> dotprod1/2, dotprod2/2, dotprod3/2, dotprod4/2, dotprod5/2, dotprod6/2, dotprod7/2, dotprod8/2, dotprod9/2, dotprod10/2
  dotprod1/1 -> Mux/1
  "IW{4,3}(2,:)'"/1 -> dotprod2/1
  dotprod2/1 -> Mux/2
  "IW{4,3}(3,:)'"/1 -> dotprod3/1
  dotprod3/1 -> Mux/3
  "IW{4,3}(4,:)'"/1 -> dotprod4/1
  dotprod4/1 -> Mux/4
  "IW{4,3}(5,:)'"/1 -> dotprod5/1
  dotprod5/1 -> Mux/5
  "IW{4,3}(6,:)'"/1 -> dotprod6/1
  dotprod6/1 -> Mux/6
  "IW{4,3}(7,:)'"/1 -> dotprod7/1
  dotprod7/1 -> Mux/7
  "IW{4,3}(8,:)'"/1 -> dotprod8/1
  dotprod8/1 -> Mux/8
  "IW{4,3}(9,:)'"/1 -> dotprod9/1
  dotprod9/1 -> Mux/9
  "IW{4,3}(10,:)'"/1 -> dotprod10/1
  dotprod10/1 -> Mux/10
  Mux/1 -> "lz{4,3}"/1

== system SC_FFNN_trainlm_10_10_10_10_Dec_8_M/Subsystem/Feed-Forward Neural Network/Layer 5/Delays 1 ==
  "p{5}" : Inport  PortDimensions=10
      mask Display: e = 0.06;c1 = [120 230 180]/255;c2 = ([120 230 180]+0)/(256+128);c3 = ([120 230 180]+128)/(256+128);patch([0 1 1 0],[0 0 1 1],c1);patch([0 1 1 1-e 1-e 0+e],[0 0 1 1-e 0+e 0+e],c2);patch([0 0 1 1-e 0+e 0+e],[0 1 1 1-e 1-e 0+e],c3);plot([0 1 1 0 0],[0 0 1 1 0]);
  mux : Mux  Inputs=1
      mask Display: e = 0.06;c1 = [120 150 230]/255;c2 = ([120 150 230]+0)/383;c3 = ([120 150 230]+128)/383;patch([0 1 1 0],[0 0 1 1],c1);patch([0 1 1 1-e 1-e 0+e],[0 0 1 1-e 0+e 0+e],c2);patch([0 0 1 1-e 0+e 0+e],[0 1 1 1-e 1-e 0+e],c3);plot([0 1 1 0 0],[0 0 1 1 0]);disp('Mux')
  "pd{5,4}" : Outport
      mask Display: e = 0.06;c1 = [120 230 180]/255;c2 = ([120 230 180]+0)/(256+128);c3 = ([120 230 180]+128)/(256+128);patch([0 1 1 0],[0 0 1 1],c1);patch([0 1 1 1-e 1-e 0+e],[0 0 1 1-e 0+e 0+e],c2);patch([0 0 1 1-e 0+e 0+e],[0 1 1 1-e 1-e 0+e],c3);plot([0 1 1 0 0],[0 0 1 1 0]);
  wires:
  "p{5}"/1 -> mux/1
  mux/1 -> "pd{5,4}"/1

== system SC_FFNN_trainlm_10_10_10_10_Dec_8_M/Subsystem/Feed-Forward Neural Network/Layer 5/LW{5,4} ==
  "ad{5,4}" : Inport  PortDimensions=10
      mask Display: e = 0.06;c1 = [120 230 180]/255;c2 = ([120 230 180]+0)/(256+128);c3 = ([120 230 180]+128)/(256+128);patch([0 1 1 0],[0 0 1 1],c1);patch([0 1 1 1-e 1-e 0+e],[0 0 1 1-e 0+e 0+e],c2);patch([0 0 1 1-e 0+e 0+e],[0 1 1 1-e 1-e 0+e],c3);plot([0 1 1 0 0],[0 0 1 1 0]);
  "IW{5,4}(1,:)'" : Constant  Value=[0.0697649567134490944386726596349035389721393585205078125;-0.88127589289447894049800424909335561096668243408203125;0.033099626411362916000857836706927628256380558013916015625;0.42375239654393592747538832554710097610950469970703125;-0.5217909805531528721900258460664190351963043212890625;0.06398832131567415426598444128103437833487987518310546875;0.09014633666209496964949465791505645029246807098388671875;-0.0027926822387992909953180475923772974056191742420196533203125;0.85925274039199150966084062019945122301578521728515625;-0.1659336458593345386969275523370015434920787811279296875]
      mask Display: e = 0.06;c1 = [120 150 230]/255;c2 = ([120 150 230]+0)/383;c3 = ([120 150 230]+128)/383;patch([0 1 1 0],[0 0 1 1],c1);patch([0 1 1 1-e 1-e 0+e],[0 0 1 1-e 0+e 0+e],c2);patch([0 0 1 1-e 0+e 0+e],[0 1 1 1-e 1-e 0+e],c3);plot([0 1 1 0 0],[0 0 1 1 0]);disp('weights');
  Mux : Mux  Inputs=1
      mask Display: e = 0.06;c1 = [120 150 230]/255;c2 = ([120 150 230]+0)/383;c3 = ([120 150 230]+128)/383;patch([0 1 1 0],[0 0 1 1],c1);patch([0 1 1 1-e 1-e 0+e],[0 0 1 1-e 0+e 0+e],c2);patch([0 0 1 1-e 0+e 0+e],[0 1 1 1-e 1-e 0+e],c3);plot([0 1 1 0 0],[0 0 1 1 0]);disp('Mux');
  dotprod1 : neural/Weight Functions/dotprod
  "lz{5,4}" : Outport
      mask Display: e = 0.06;c1 = [120 230 180]/255;c2 = ([120 230 180]+0)/(256+128);c3 = ([120 230 180]+128)/(256+128);patch([0 1 1 0],[0 0 1 1],c1);patch([0 1 1 1-e 1-e 0+e],[0 0 1 1-e 0+e 0+e],c2);patch([0 0 1 1-e 0+e 0+e],[0 1 1 1-e 1-e 0+e],c3);plot([0 1 1 0 0],[0 0 1 1 0]);
  wires:
  "IW{5,4}(1,:)'"/1 -> dotprod1/1
  "ad{5,4}"/1 -> dotprod1/2
  dotprod1/1 -> Mux/1
  Mux/1 -> "lz{5,4}"/1
